simulink model "ANS_GFM_short_term"  (R2021b)
settings: Solver=FixedStepAuto  StartTime=0.0  StopTime=5  FixedStep=Ts  MaxStep=1e-5  RelTol=1e-3
values from neighbouring files (symbols this model uses):
  angle_load = angle(LF.bus(ind_l).Vbus)*180/pi    [init_ANS_GFM_long_term.m]    (also in init_ANS_GFM_short_term.m)
  angleV_LF = Vangle_init/180*pi    [init_ANS_GFM_long_term.m]    (also in init_ANS_GFM_short_term.m)
  awu = 1    [init_ANS_GFM_long_term.m]    (also in init_ANS_GFM_short_term.m)
  C_dc = 1/(Xcdc_pu_or*Zbase_dc_new*100*pi)    [init_ANS_GFM_long_term.m]    (also in init_ANS_GFM_short_term.m)
  C_f = 1/(Xcf_pu_or*Zbase_new*100*pi)    (= 0.013712)    [init_ANS_GFM_long_term.m]    (also in init_ANS_GFM_short_term.m = 0.0141333333333)
  control = 3    [init_ANS_GFM_long_term.m]    (also in init_ANS_GFM_short_term.m = 1)
  D_p = (1/(m_p*w_b))    (= 5209935.26289)    [init_ANS_GFM_long_term.m]    (also in init_ANS_GFM_short_term.m = 5370022.73304)
  Egrid_tmp = 1.054080675694902*400e3    (= 421632.270278)    [init_ANS_GFM_long_term.m]    (also in init_ANS_GFM_short_term.m)
  epsi = 1e-4    (= 0.0001)    [init_ANS_GFM_long_term.m]    (also in init_ANS_GFM_short_term.m)
  eta = m_p*V_m^2    [init_ANS_GFM_long_term.m]    (also in init_ANS_GFM_short_term.m)
  gamma = 2.3    [init_ANS_GFM_long_term.m]    (also in init_ANS_GFM_short_term.m)
  I0_init = [I0_init_a, I0_init_b, I0_init_c]    [init_ANS_GFM_long_term.m]    (also in init_ANS_GFM_short_term.m)
  I_bc = S_bc / (V_bc*sqrt(3))    [init_ANS_GFM_long_term.m]    (also in init_ANS_GFM_short_term.m)
  I_d_int_init = (U_d_int + I_q_int*L_f*w_b - V_d_int - I_d_int*R_f*0)    [init_ANS_GFM_long_term.m]    (also in init_ANS_GFM_short_term.m)
  I_init = [I_init_a, I_init_b, I_init_c]    [init_ANS_GFM_long_term.m]    (also in init_ANS_GFM_short_term.m)
  i_ll = -1.15*(S_bc/Vdc_n)-i_loss_dc    [init_ANS_GFM_long_term.m]    (also in init_ANS_GFM_short_term.m)
  I_max_sat_pu = 1.0 * I_bc *sqrt(2)    [init_ANS_GFM_long_term.m]    (also in init_ANS_GFM_short_term.m)
  I_q_int_init = (U_q_int - I_d_int*L_f*w_b - V_q_int - I_q_int*R_f*0)    [init_ANS_GFM_long_term.m]    (also in init_ANS_GFM_short_term.m)
  i_ul = 1.15*(S_bc/Vdc_n)+i_loss_dc    [init_ANS_GFM_long_term.m]    (also in init_ANS_GFM_short_term.m)
  idppu = 0.95    [init_ANS_GFM_long_term.m]    (also in init_ANS_GFM_short_term.m = 0.92)
  init_dP = -inv(A_pm)*B_pm*dP    [init_ANS_GFM_long_term.m]    (also in init_ANS_GFM_short_term.m)
  init_pm = -inv(A_pm)*B_pm*P_aft    [init_ANS_GFM_long_term.m]    (also in init_ANS_GFM_short_term.m)
  init_tau = -inv(A_tau)*B_tau*idc    [init_ANS_GFM_long_term.m]    (also in init_ANS_GFM_short_term.m)
  J = D_p*tau_f    (= 104198.705258)    [init_ANS_GFM_long_term.m]    (also in init_ANS_GFM_short_term.m = 107400.454661)
  k_dc = eta_1/(Vdc_n*m_p)    [init_ANS_GFM_long_term.m]    (also in init_ANS_GFM_short_term.m)
  K_p = (1/Vdc_n)    [init_ANS_GFM_long_term.m]    (also in init_ANS_GFM_short_term.m)
  K_r = 1/R_dc    [init_ANS_GFM_long_term.m]    (also in init_ANS_GFM_short_term.m)
  Kff_i = 1    [init_ANS_GFM_long_term.m]    (also in init_ANS_GFM_short_term.m)
  Kff_v = 1    [init_ANS_GFM_long_term.m]    (also in init_ANS_GFM_short_term.m)
  Ki_i = (1/n)*1.19    (= 0.0520711785298)    [init_ANS_GFM_long_term.m]    (also in init_ANS_GFM_short_term.m = 0.0505188679245)
  Ki_pll = 4255.3    [init_ANS_GFM_long_term.m]    (also in init_ANS_GFM_short_term.m)
  Ki_v = (n)*1.161022    (= 26.5332227733)    [init_ANS_GFM_long_term.m]    (also in init_ANS_GFM_short_term.m = 27.3485182222)
  ki_v_ac = 2*0.25    (= 0.5)    [init_ANS_GFM_long_term.m]    (also in init_ANS_GFM_short_term.m)
  Kp_i = 0.738891/n    (= 0.032331869895)    [init_ANS_GFM_long_term.m]    (also in init_ANS_GFM_short_term.m = 0.0313680141509)
  Kp_pll = 92    [init_ANS_GFM_long_term.m]    (also in init_ANS_GFM_short_term.m)
  Kp_v = 0.52*n    (= 11.8837333333)    [init_ANS_GFM_long_term.m]    (also in init_ANS_GFM_short_term.m = 12.2488888889)
  kp_v_ac = 0.001    [init_ANS_GFM_long_term.m]    (also in init_ANS_GFM_short_term.m)
  Kpl = 5.0    (= 5)    [init_ANS_GFM_long_term.m]    (also in init_ANS_GFM_short_term.m)
  L1 = cf/sqrt(1+RX^2)*(400e3)^2/Skss/(100*pi)    [init_ANS_GFM_long_term.m]    (also in init_ANS_GFM_short_term.m)
  L_f = Xlf_pu_or*Zbase_new/100/pi    (= 4.37572928821e-06)    [init_ANS_GFM_long_term.m]    (also in init_ANS_GFM_short_term.m = 4.24528301887e-06)
  Lf = 1e6/100/pi    (= 3183.09886184)    [init_ANS_GFM_long_term.m]    (also in init_ANS_GFM_short_term.m = 0.0636619772368)
  m_p = (2*pi*0.5)/(S_bc)    (= 6.10967066042e-10)    [init_ANS_GFM_long_term.m]    (also in init_ANS_GFM_short_term.m = 5.92753330866e-10)
  n = 1/Zb    (= 22.8533333333)    [init_ANS_GFM_long_term.m]    (also in init_ANS_GFM_short_term.m = 23.5555555556)
  P_LF_si = P_LF*S_b    [init_ANS_GFM_long_term.m]    (also in init_ANS_GFM_short_term.m)
  ps = 4440e6/S_bc    (= 0.863477246208)    [init_ANS_GFM_long_term.m]    (also in init_ANS_GFM_short_term.m = 0.837735849057)
  Q_LF_si = Q_LF*S_b    [init_ANS_GFM_long_term.m]    (also in init_ANS_GFM_short_term.m)
  qs = Q_LF*S_b/S_bc    [init_ANS_GFM_long_term.m]    (also in init_ANS_GFM_short_term.m)
  R1 = RX*cf/sqrt(1+RX^2)*(400e3)^2/Skss    [init_ANS_GFM_long_term.m]    (also in init_ANS_GFM_short_term.m)
  R_dc = Rdc_pu_or*Zbase_dc_new    [init_ANS_GFM_long_term.m]    (also in init_ANS_GFM_short_term.m)
  R_f = Rf_pu_or*Zbase_new    (= 2.18786464411e-05)    [init_ANS_GFM_long_term.m]    (also in init_ANS_GFM_short_term.m = 2.12264150943e-05)
  Rf = 1e6    (= 1000000)    [init_ANS_GFM_long_term.m]    (also in init_ANS_GFM_short_term.m = 20)
  S_bc = 5142e6    (= 5142000000)    [init_ANS_GFM_long_term.m]    (also in init_ANS_GFM_short_term.m = 5300000000)
  sat_select = 3    [init_ANS_GFM_long_term.m]    (also in init_ANS_GFM_short_term.m)
  SECM = 3    [init_ANS_GFM_long_term.m]    (also in init_ANS_GFM_short_term.m = 1)
  share_i_load = 1.0    (= 1)    [init_ANS_GFM_long_term.m]    (also in init_ANS_GFM_short_term.m)
  T_en = -0.5    [init_ANS_GFM_long_term.m]    (also in init_ANS_GFM_short_term.m)
  T_off = T_on + 0.1    (= 0.2)    [init_ANS_GFM_long_term.m]    (also in init_ANS_GFM_short_term.m)
  T_on = 0.1    [init_ANS_GFM_long_term.m]    (also in init_ANS_GFM_short_term.m)
  Ts = 2e-6    (= 2e-06)    [init_ANS_GFM_long_term.m]    (also in init_ANS_GFM_short_term.m = 1e-06)
  U_init = [Umag_init_a, Umag_init_b, Umag_init_c]    [init_ANS_GFM_long_term.m]    (also in init_ANS_GFM_short_term.m)
  Uangle_init = angle(V_LF_VSC)*180/pi    [init_ANS_GFM_long_term.m]    (also in init_ANS_GFM_short_term.m)
  Umag_init = abs(V_LF_VSC)*V_bc*sqrt(2/3)    [init_ANS_GFM_long_term.m]    (also in init_ANS_GFM_short_term.m)
  V1_rms = 15e3    (= 15000)    [init_ANS_GFM_long_term.m]    (also in init_ANS_GFM_short_term.m)
  V_d_int = abs(V_LF)*V_bc*sqrt(2/3)    [init_ANS_GFM_long_term.m]    (also in init_ANS_GFM_short_term.m)
  V_d_int_init = (I_d_int + V_q_int*C_f*w_b - I0_d_int)    [init_ANS_GFM_long_term.m]    (also in init_ANS_GFM_short_term.m)
  V_init = [V_init_a, V_init_b, V_init_c]    [init_ANS_GFM_long_term.m]    (also in init_ANS_GFM_short_term.m)
  V_m = sqrt(2/3)*V_bc    [init_ANS_GFM_long_term.m]    (also in init_ANS_GFM_short_term.m)
  V_q_int_init = (I_q_int - V_d_int*C_f*w_b - I0_q_int)    [init_ANS_GFM_long_term.m]    (also in init_ANS_GFM_short_term.m)
  Vdc_n = 3*V_m    [init_ANS_GFM_long_term.m]    (also in init_ANS_GFM_short_term.m)
  Vref = V_LF_mag*V_m    [init_ANS_GFM_long_term.m]    (also in init_ANS_GFM_short_term.m)
  w_b = 2*pi*f_b    (= 314.159265359)    [init_ANS_GFM_long_term.m]    (also in init_ANS_GFM_short_term.m)
  w_f = 2*pi*5    (= 31.4159265359)    [init_ANS_GFM_long_term.m]    (also in init_ANS_GFM_short_term.m)
  Zbase_new = V1_rms^2/S_bc    (= 0.0437572928821)    [init_ANS_GFM_long_term.m]    (also in init_ANS_GFM_short_term.m = 0.0424528301887)
undefined symbols (not defined in the file or in its folder): A_pm, A_tau, B_pm, B_tau, C_pm, C_tau, D_pm, D_tau, find_system, idq0_init, Pm, sm_init, v_d, v_q, Ve
libraries: spsBreakerLib x270, spsGroundLib x21, spsThreePhaseSeriesRLCBranchLib x12, spsabctodq0Lib x11, simulink x9, spsEdgeDetectorLib x8, spsThreePhaseVIMeasurementLib x7, spsLoadFlowBusLib x7, spsSeriesRLCBranchLib x6, spsControlledVoltageSourceLib x6, spsCurrentMeasurementLib x6, spsVoltageMeasurementLib x6
(part 4 of 7)

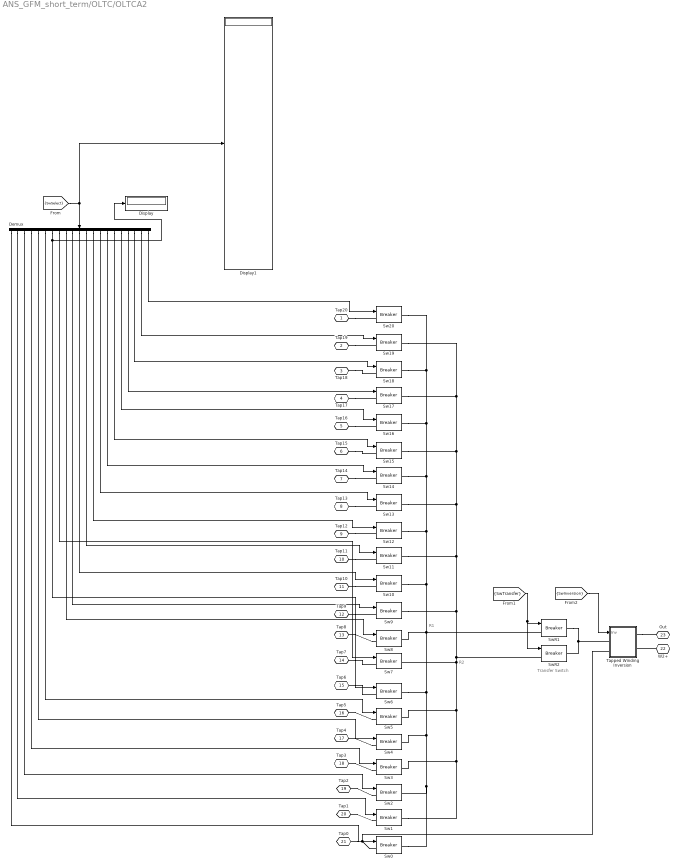
== system ANS_GFM_short_term/OLTC/OLTCA2 ==
  note: R2
  note: R1
  note: Transfer Switch
  Demux : Demux  Outputs=21
      settings: DisplayOption=none
  Display : Display
  Display1 : Display
  "Sw0 " : spsBreakerLib/Breaker  InitialState=InitialStates(1)  SwitchingTimes="[ 1/60  5/60 ]"  External=on  BreakerResistance=Rswitch  SnubberResistance=1e8  SnubberCapacitance=inf  Measurements=None  MoreParameters=off  NoBreakLoop=off
      settings: SourceProductBaseCode=PS
  "Sw1 " : spsBreakerLib/Breaker  InitialState=InitialStates(2)  SwitchingTimes="[ 1/60  5/60 ]"  External=on  BreakerResistance=Rswitch  SnubberResistance=1e8  SnubberCapacitance=inf  Measurements=None  MoreParameters=off  NoBreakLoop=off
      settings: SourceProductBaseCode=PS
  Sw10 : spsBreakerLib/Breaker  InitialState=InitialStates(11)  SwitchingTimes="[ 1/60  5/60 ]"  External=on  BreakerResistance=Rswitch  SnubberResistance=1e8  SnubberCapacitance=inf  Measurements=None  MoreParameters=off  NoBreakLoop=off
      settings: SourceProductBaseCode=PS
  Sw11 : spsBreakerLib/Breaker  InitialState=InitialStates(12)  SwitchingTimes="[ 1/60  5/60 ]"  External=on  BreakerResistance=Rswitch  SnubberResistance=1e8  SnubberCapacitance=inf  Measurements=None  MoreParameters=off  NoBreakLoop=off
      settings: SourceProductBaseCode=PS
  Sw12 : spsBreakerLib/Breaker  InitialState=InitialStates(13)  SwitchingTimes="[ 1/60  5/60 ]"  External=on  BreakerResistance=Rswitch  SnubberResistance=1e8  SnubberCapacitance=inf  Measurements=None  MoreParameters=off  NoBreakLoop=off
      settings: SourceProductBaseCode=PS
  Sw13 : spsBreakerLib/Breaker  InitialState=InitialStates(14)  SwitchingTimes="[ 1/60  5/60 ]"  External=on  BreakerResistance=Rswitch  SnubberResistance=1e8  SnubberCapacitance=inf  Measurements=None  MoreParameters=off  NoBreakLoop=off
      settings: SourceProductBaseCode=PS
  Sw14 : spsBreakerLib/Breaker  InitialState=InitialStates(15)  SwitchingTimes="[ 1/60  5/60 ]"  External=on  BreakerResistance=Rswitch  SnubberResistance=1e8  SnubberCapacitance=inf  Measurements=None  MoreParameters=off  NoBreakLoop=off
      settings: SourceProductBaseCode=PS
  Sw15 : spsBreakerLib/Breaker  InitialState=InitialStates(16)  SwitchingTimes="[ 1/60  5/60 ]"  External=on  BreakerResistance=Rswitch  SnubberResistance=1e8  SnubberCapacitance=inf  Measurements=None  MoreParameters=off  NoBreakLoop=off
      settings: SourceProductBaseCode=PS
  Sw16 : spsBreakerLib/Breaker  InitialState=InitialStates(17)  SwitchingTimes="[ 1/60  5/60 ]"  External=on  BreakerResistance=Rswitch  SnubberResistance=1e8  SnubberCapacitance=inf  Measurements=None  MoreParameters=off  NoBreakLoop=off
      settings: SourceProductBaseCode=PS
  Sw17 : spsBreakerLib/Breaker  InitialState=InitialStates(18)  SwitchingTimes="[ 1/60  5/60 ]"  External=on  BreakerResistance=Rswitch  SnubberResistance=1e8  SnubberCapacitance=inf  Measurements=None  MoreParameters=off  NoBreakLoop=off
      settings: SourceProductBaseCode=PS
  Sw18 : spsBreakerLib/Breaker  InitialState=InitialStates(19)  SwitchingTimes="[ 1/60  5/60 ]"  External=on  BreakerResistance=Rswitch  SnubberResistance=1e8  SnubberCapacitance=inf  Measurements=None  MoreParameters=off  NoBreakLoop=off
      settings: SourceProductBaseCode=PS
  Sw19 : spsBreakerLib/Breaker  InitialState=InitialStates(20)  SwitchingTimes="[ 1/60  5/60 ]"  External=on  BreakerResistance=Rswitch  SnubberResistance=1e8  SnubberCapacitance=inf  Measurements=None  MoreParameters=off  NoBreakLoop=off
      settings: SourceProductBaseCode=PS
  "Sw2 " : spsBreakerLib/Breaker  InitialState=InitialStates(3)  SwitchingTimes="[ 1/60  5/60 ]"  External=on  BreakerResistance=Rswitch  SnubberResistance=1e8  SnubberCapacitance=inf  Measurements=None  MoreParameters=off  NoBreakLoop=off
      settings: SourceProductBaseCode=PS
  Sw20 : spsBreakerLib/Breaker  InitialState=InitialStates(21)  SwitchingTimes="[ 1/60  5/60 ]"  External=on  BreakerResistance=Rswitch  SnubberResistance=Rsnubber  SnubberCapacitance=inf  Measurements=None  MoreParameters=off  NoBreakLoop=off
      settings: SourceProductBaseCode=PS
  "Sw3 " : spsBreakerLib/Breaker  InitialState=InitialStates(4)  SwitchingTimes="[ 1/60  5/60 ]"  External=on  BreakerResistance=Rswitch  SnubberResistance=1e8  SnubberCapacitance=inf  Measurements=None  MoreParameters=off  NoBreakLoop=off
      settings: SourceProductBaseCode=PS
  "Sw4 " : spsBreakerLib/Breaker  InitialState=InitialStates(5)  SwitchingTimes="[ 1/60  5/60 ]"  External=on  BreakerResistance=Rswitch  SnubberResistance=1e8  SnubberCapacitance=inf  Measurements=None  MoreParameters=off  NoBreakLoop=off
      settings: SourceProductBaseCode=PS
  "Sw5 " : spsBreakerLib/Breaker  InitialState=InitialStates(6)  SwitchingTimes="[ 1/60  5/60 ]"  External=on  BreakerResistance=Rswitch  SnubberResistance=1e8  SnubberCapacitance=inf  Measurements=None  MoreParameters=off  NoBreakLoop=off
      settings: SourceProductBaseCode=PS
  "Sw6 " : spsBreakerLib/Breaker  InitialState=InitialStates(7)  SwitchingTimes="[ 1/60  5/60 ]"  External=on  BreakerResistance=Rswitch  SnubberResistance=1e8  SnubberCapacitance=inf  Measurements=None  MoreParameters=off  NoBreakLoop=off
      settings: SourceProductBaseCode=PS
  "Sw7 " : spsBreakerLib/Breaker  InitialState=InitialStates(8)  SwitchingTimes="[ 1/60  5/60 ]"  External=on  BreakerResistance=Rswitch  SnubberResistance=1e8  SnubberCapacitance=inf  Measurements=None  MoreParameters=off  NoBreakLoop=off
      settings: SourceProductBaseCode=PS
  "Sw8 " : spsBreakerLib/Breaker  InitialState=InitialStates(9)  SwitchingTimes="[ 1/60  5/60 ]"  External=on  BreakerResistance=Rswitch  SnubberResistance=1e8  SnubberCapacitance=inf  Measurements=None  MoreParameters=off  NoBreakLoop=off
      settings: SourceProductBaseCode=PS
  Sw9 : spsBreakerLib/Breaker  InitialState=InitialStates(10)  SwitchingTimes="[ 1/60  5/60 ]"  External=on  BreakerResistance=Rswitch  SnubberResistance=1e8  SnubberCapacitance=inf  Measurements=None  MoreParameters=off  NoBreakLoop=off
      settings: SourceProductBaseCode=PS
  SwR1 : spsBreakerLib/Breaker  InitialState=1  SwitchingTimes="[ 1/60  5/60 ]"  External=on  BreakerResistance=Rswitch  SnubberResistance=Rtransfer  SnubberCapacitance=inf  Measurements=None  MoreParameters=off  NoBreakLoop=off
      settings: SourceProductBaseCode=PS
  SwR2 : spsBreakerLib/Breaker  InitialState=1  SwitchingTimes="[ 1/60  5/60 ]"  External=on  BreakerResistance=Rswitch  SnubberResistance=Rtransfer  SnubberCapacitance=inf  Measurements=None  MoreParameters=off  NoBreakLoop=off
      settings: SourceProductBaseCode=PS
  Tapped Winding Inversion : Subsystem
  Tap20 : PMIOPort  Side=Right
  Tap19 : PMIOPort  Port=2  Side=Right
  Tap18 : PMIOPort  Port=3  Side=Right
  Tap17 : PMIOPort  Port=4  Side=Right
  Tap16 : PMIOPort  Port=5  Side=Right
  Tap15 : PMIOPort  Port=6  Side=Right
  Tap14 : PMIOPort  Port=7  Side=Right
  Tap13 : PMIOPort  Port=8  Side=Right
  Tap12 : PMIOPort  Port=9  Side=Right
  Tap11 : PMIOPort  Port=10  Side=Right
  Tap10 : PMIOPort  Port=11  Side=Right
  Tap9 : PMIOPort  Port=12  Side=Right
  Tap8 : PMIOPort  Port=13  Side=Right
  Tap7 : PMIOPort  Port=14  Side=Right
  Tap6 : PMIOPort  Port=15  Side=Right
  Tap5 : PMIOPort  Port=16  Side=Right
  Tap4 : PMIOPort  Port=17  Side=Right
  Tap3 : PMIOPort  Port=18  Side=Right
  Tap2 : PMIOPort  Port=19  Side=Right
  Tap1 : PMIOPort  Port=20  Side=Right
  Tap0 : PMIOPort  Port=21  Side=Right
  W2+ : PMIOPort  Port=22  Side=Right
  Out : PMIOPort  Port=23  Side=Left
  wires:
  Demux/9 -> "Sw8 "/1
  Demux/8 -> "Sw7 "/1
  Demux/7 -> Display/1, "Sw6 "/1
  Demux/6 -> "Sw5 "/1
  Demux/5 -> "Sw4 "/1
  Demux/4 -> "Sw3 "/1
  Demux/3 -> "Sw2 "/1
  Demux/2 -> "Sw1 "/1
  Demux/1 -> "Sw0 "/1
  [SwInversion] -> Tapped Winding Inversion/1(Inv)
  [SwTransfer] -> SwR2/1, SwR1/1
  [SwSelect] -> Demux/1, Display1/1
  Demux/10 -> Sw9/1
  Demux/11 -> Sw10/1
  Demux/12 -> Sw11/1
  Demux/13 -> Sw12/1
  Demux/14 -> Sw13/1
  Demux/15 -> Sw14/1
  Demux/16 -> Sw15/1
  Demux/17 -> Sw16/1
  Demux/18 -> Sw17/1
  Demux/19 -> Sw18/1
  Demux/20 -> Sw19/1
  Demux/21 -> Sw20/1
  connections:
  "Sw0 "/LConn1 -- Tap0/RConn1 -- Tapped Winding Inversion/LConn2
  Tap1/RConn1 -- "Sw1 "/LConn1
  Tap2/RConn1 -- "Sw2 "/LConn1
  Tap6/RConn1 -- "Sw6 "/LConn1
  Tap4/RConn1 -- "Sw4 "/LConn1
  Tap5/RConn1 -- "Sw5 "/LConn1
  SwR1/RConn1 -- Tapped Winding Inversion/LConn1 -- SwR2/RConn1
  Sw19/RConn1 -- Sw17/RConn1 -- Sw15/RConn1 -- Sw13/RConn1 -- Sw11/RConn1 -- Sw9/RConn1 -- SwR2/LConn1 -- "Sw5 "/RConn1 -- "Sw3 "/RConn1 -- "Sw1 "/RConn1 -- "Sw7 "/RConn1
  Tapped Winding Inversion/RConn1 -- Out/RConn1
  W2+/RConn1 -- Tapped Winding Inversion/RConn2
  "Sw6 "/RConn1 -- "Sw4 "/RConn1 -- "Sw2 "/RConn1 -- "Sw0 "/RConn1 -- Sw20/RConn1 -- Sw18/RConn1 -- Sw16/RConn1 -- Sw14/RConn1 -- Sw12/RConn1 -- Sw10/RConn1 -- "Sw8 "/RConn1 -- SwR1/LConn1
  Tap3/RConn1 -- "Sw3 "/LConn1
  Tap8/RConn1 -- "Sw8 "/LConn1
  Tap7/RConn1 -- "Sw7 "/LConn1
  Tap9/RConn1 -- Sw9/LConn1
  Tap10/RConn1 -- Sw10/LConn1
  Tap11/RConn1 -- Sw11/LConn1
  Tap13/RConn1 -- Sw13/LConn1
  Tap12/RConn1 -- Sw12/LConn1
  Tap14/RConn1 -- Sw14/LConn1
  Tap15/RConn1 -- Sw15/LConn1
  Tap16/RConn1 -- Sw16/LConn1
  Tap17/RConn1 -- Sw17/LConn1
  Tap18/RConn1 -- Sw18/LConn1
  Tap19/RConn1 -- Sw19/LConn1
  Tap20/RConn1 -- Sw20/LConn1

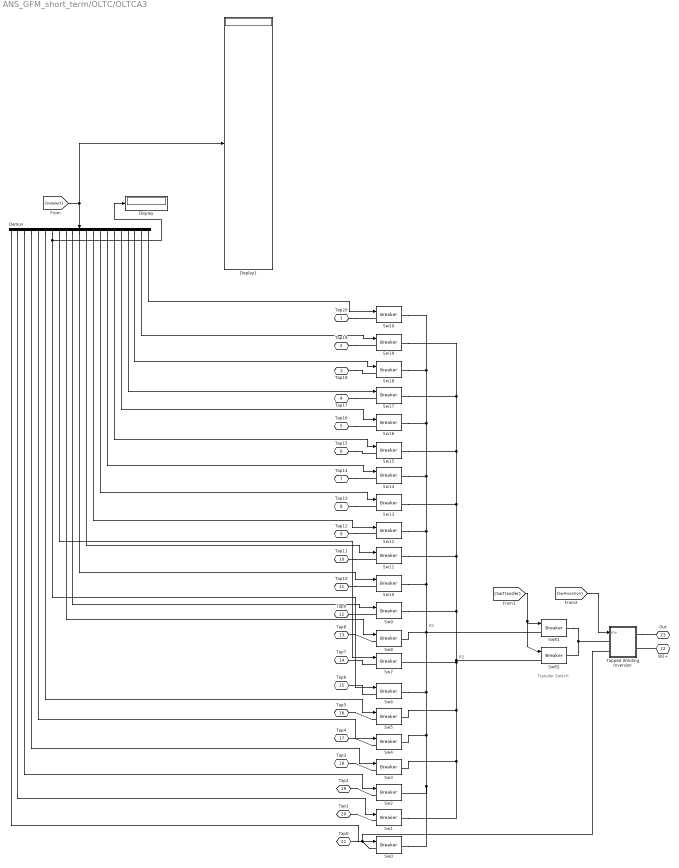
== system ANS_GFM_short_term/OLTC/OLTCA3 ==
  note: R2
  note: R1
  note: Transfer Switch
  Demux : Demux  Outputs=21
      settings: DisplayOption=none
  Display : Display
  Display1 : Display
  "Sw0 " : spsBreakerLib/Breaker  InitialState=InitialStates(1)  SwitchingTimes="[ 1/60  5/60 ]"  External=on  BreakerResistance=1e-8  SnubberResistance=1e8  SnubberCapacitance=inf  Measurements=None  MoreParameters=off  NoBreakLoop=off
      settings: SourceProductBaseCode=PS
  "Sw1 " : spsBreakerLib/Breaker  InitialState=InitialStates(2)  SwitchingTimes="[ 1/60  5/60 ]"  External=on  BreakerResistance=1e-8  SnubberResistance=1e8  SnubberCapacitance=inf  Measurements=None  MoreParameters=off  NoBreakLoop=off
      settings: SourceProductBaseCode=PS
  Sw10 : spsBreakerLib/Breaker  InitialState=InitialStates(11)  SwitchingTimes="[ 1/60  5/60 ]"  External=on  BreakerResistance=1e-8  SnubberResistance=1e8  SnubberCapacitance=inf  Measurements=None  MoreParameters=off  NoBreakLoop=off
      settings: SourceProductBaseCode=PS
  Sw11 : spsBreakerLib/Breaker  InitialState=InitialStates(12)  SwitchingTimes="[ 1/60  5/60 ]"  External=on  BreakerResistance=1e-8  SnubberResistance=1e8  SnubberCapacitance=inf  Measurements=None  MoreParameters=off  NoBreakLoop=off
      settings: SourceProductBaseCode=PS
  Sw12 : spsBreakerLib/Breaker  InitialState=InitialStates(13)  SwitchingTimes="[ 1/60  5/60 ]"  External=on  BreakerResistance=1e-8  SnubberResistance=1e8  SnubberCapacitance=inf  Measurements=None  MoreParameters=off  NoBreakLoop=off
      settings: SourceProductBaseCode=PS
  Sw13 : spsBreakerLib/Breaker  InitialState=InitialStates(14)  SwitchingTimes="[ 1/60  5/60 ]"  External=on  BreakerResistance=1e-8  SnubberResistance=1e8  SnubberCapacitance=inf  Measurements=None  MoreParameters=off  NoBreakLoop=off
      settings: SourceProductBaseCode=PS
  Sw14 : spsBreakerLib/Breaker  InitialState=InitialStates(15)  SwitchingTimes="[ 1/60  5/60 ]"  External=on  BreakerResistance=1e-8  SnubberResistance=1e8  SnubberCapacitance=inf  Measurements=None  MoreParameters=off  NoBreakLoop=off
      settings: SourceProductBaseCode=PS
  Sw15 : spsBreakerLib/Breaker  InitialState=InitialStates(16)  SwitchingTimes="[ 1/60  5/60 ]"  External=on  BreakerResistance=1e-8  SnubberResistance=1e8  SnubberCapacitance=inf  Measurements=None  MoreParameters=off  NoBreakLoop=off
      settings: SourceProductBaseCode=PS
  Sw16 : spsBreakerLib/Breaker  InitialState=InitialStates(17)  SwitchingTimes="[ 1/60  5/60 ]"  External=on  BreakerResistance=1e-8  SnubberResistance=1e8  SnubberCapacitance=inf  Measurements=None  MoreParameters=off  NoBreakLoop=off
      settings: SourceProductBaseCode=PS
  Sw17 : spsBreakerLib/Breaker  InitialState=InitialStates(18)  SwitchingTimes="[ 1/60  5/60 ]"  External=on  BreakerResistance=1e-8  SnubberResistance=1e8  SnubberCapacitance=inf  Measurements=None  MoreParameters=off  NoBreakLoop=off
      settings: SourceProductBaseCode=PS
  Sw18 : spsBreakerLib/Breaker  InitialState=InitialStates(19)  SwitchingTimes="[ 1/60  5/60 ]"  External=on  BreakerResistance=1e-8  SnubberResistance=1e8  SnubberCapacitance=inf  Measurements=None  MoreParameters=off  NoBreakLoop=off
      settings: SourceProductBaseCode=PS
  Sw19 : spsBreakerLib/Breaker  InitialState=InitialStates(20)  SwitchingTimes="[ 1/60  5/60 ]"  External=on  BreakerResistance=1e-8  SnubberResistance=1e8  SnubberCapacitance=inf  Measurements=None  MoreParameters=off  NoBreakLoop=off
      settings: SourceProductBaseCode=PS
  "Sw2 " : spsBreakerLib/Breaker  InitialState=InitialStates(3)  SwitchingTimes="[ 1/60  5/60 ]"  External=on  BreakerResistance=1e-8  SnubberResistance=1e8  SnubberCapacitance=inf  Measurements=None  MoreParameters=off  NoBreakLoop=off
      settings: SourceProductBaseCode=PS
  Sw20 : spsBreakerLib/Breaker  InitialState=InitialStates(21)  SwitchingTimes="[ 1/60  5/60 ]"  External=on  BreakerResistance=1e-8  SnubberResistance=1e8  SnubberCapacitance=inf  Measurements=None  MoreParameters=off  NoBreakLoop=off
      settings: SourceProductBaseCode=PS
  "Sw3 " : spsBreakerLib/Breaker  InitialState=InitialStates(4)  SwitchingTimes="[ 1/60  5/60 ]"  External=on  BreakerResistance=1e-8  SnubberResistance=1e8  SnubberCapacitance=inf  Measurements=None  MoreParameters=off  NoBreakLoop=off
      settings: SourceProductBaseCode=PS
  "Sw4 " : spsBreakerLib/Breaker  InitialState=InitialStates(5)  SwitchingTimes="[ 1/60  5/60 ]"  External=on  BreakerResistance=1e-8  SnubberResistance=1e8  SnubberCapacitance=inf  Measurements=None  MoreParameters=off  NoBreakLoop=off
      settings: SourceProductBaseCode=PS
  "Sw5 " : spsBreakerLib/Breaker  InitialState=InitialStates(6)  SwitchingTimes="[ 1/60  5/60 ]"  External=on  BreakerResistance=1e-8  SnubberResistance=1e8  SnubberCapacitance=inf  Measurements=None  MoreParameters=off  NoBreakLoop=off
      settings: SourceProductBaseCode=PS
  "Sw6 " : spsBreakerLib/Breaker  InitialState=InitialStates(7)  SwitchingTimes="[ 1/60  5/60 ]"  External=on  BreakerResistance=1e-8  SnubberResistance=1e8  SnubberCapacitance=inf  Measurements=None  MoreParameters=off  NoBreakLoop=off
      settings: SourceProductBaseCode=PS
  "Sw7 " : spsBreakerLib/Breaker  InitialState=InitialStates(8)  SwitchingTimes="[ 1/60  5/60 ]"  External=on  BreakerResistance=1e-8  SnubberResistance=1e8  SnubberCapacitance=inf  Measurements=None  MoreParameters=off  NoBreakLoop=off
      settings: SourceProductBaseCode=PS
  "Sw8 " : spsBreakerLib/Breaker  InitialState=InitialStates(9)  SwitchingTimes="[ 1/60  5/60 ]"  External=on  BreakerResistance=1e-8  SnubberResistance=1e8  SnubberCapacitance=inf  Measurements=None  MoreParameters=off  NoBreakLoop=off
      settings: SourceProductBaseCode=PS
  Sw9 : spsBreakerLib/Breaker  InitialState=InitialStates(10)  SwitchingTimes="[ 1/60  5/60 ]"  External=on  BreakerResistance=1e-8  SnubberResistance=1e8  SnubberCapacitance=inf  Measurements=None  MoreParameters=off  NoBreakLoop=off
      settings: SourceProductBaseCode=PS
  SwR1 : spsBreakerLib/Breaker  InitialState=1  SwitchingTimes="[ 1/60  5/60 ]"  External=on  BreakerResistance=1e-8  SnubberResistance=Rtransfer  SnubberCapacitance=inf  Measurements=None  MoreParameters=off  NoBreakLoop=off
      settings: SourceProductBaseCode=PS
  SwR2 : spsBreakerLib/Breaker  InitialState=1  SwitchingTimes="[ 1/60  5/60 ]"  External=on  BreakerResistance=1e-8  SnubberResistance=Rtransfer  SnubberCapacitance=inf  Measurements=None  MoreParameters=off  NoBreakLoop=off
      settings: SourceProductBaseCode=PS
  Tapped Winding Inversion : Subsystem
  Tap20 : PMIOPort  Side=Right
  Tap19 : PMIOPort  Port=2  Side=Right
  Tap18 : PMIOPort  Port=3  Side=Right
  Tap17 : PMIOPort  Port=4  Side=Right
  Tap16 : PMIOPort  Port=5  Side=Right
  Tap15 : PMIOPort  Port=6  Side=Right
  Tap14 : PMIOPort  Port=7  Side=Right
  Tap13 : PMIOPort  Port=8  Side=Right
  Tap12 : PMIOPort  Port=9  Side=Right
  Tap11 : PMIOPort  Port=10  Side=Right
  Tap10 : PMIOPort  Port=11  Side=Right
  Tap9 : PMIOPort  Port=12  Side=Right
  Tap8 : PMIOPort  Port=13  Side=Right
  Tap7 : PMIOPort  Port=14  Side=Right
  Tap6 : PMIOPort  Port=15  Side=Right
  Tap5 : PMIOPort  Port=16  Side=Right
  Tap4 : PMIOPort  Port=17  Side=Right
  Tap3 : PMIOPort  Port=18  Side=Right
  Tap2 : PMIOPort  Port=19  Side=Right
  Tap1 : PMIOPort  Port=20  Side=Right
  Tap0 : PMIOPort  Port=21  Side=Right
  W2+ : PMIOPort  Port=22  Side=Right
  Out : PMIOPort  Port=23  Side=Left
  wires:
  Demux/9 -> "Sw8 "/1
  Demux/8 -> "Sw7 "/1
  Demux/7 -> Display/1, "Sw6 "/1
  Demux/6 -> "Sw5 "/1
  Demux/5 -> "Sw4 "/1
  Demux/4 -> "Sw3 "/1
  Demux/3 -> "Sw2 "/1
  Demux/2 -> "Sw1 "/1
  Demux/1 -> "Sw0 "/1
  [SwInversion] -> Tapped Winding Inversion/1(Inv)
  [SwTransfer] -> SwR2/1, SwR1/1
  [SwSelect] -> Demux/1, Display1/1
  Demux/10 -> Sw9/1
  Demux/11 -> Sw10/1
  Demux/12 -> Sw11/1
  Demux/13 -> Sw12/1
  Demux/14 -> Sw13/1
  Demux/15 -> Sw14/1
  Demux/16 -> Sw15/1
  Demux/17 -> Sw16/1
  Demux/18 -> Sw17/1
  Demux/19 -> Sw18/1
  Demux/20 -> Sw19/1
  Demux/21 -> Sw20/1
  connections:
  "Sw0 "/LConn1 -- Tap0/RConn1 -- Tapped Winding Inversion/LConn2
  Tap1/RConn1 -- "Sw1 "/LConn1
  Tap2/RConn1 -- "Sw2 "/LConn1
  Tap6/RConn1 -- "Sw6 "/LConn1
  Tap4/RConn1 -- "Sw4 "/LConn1
  Tap5/RConn1 -- "Sw5 "/LConn1
  SwR1/RConn1 -- Tapped Winding Inversion/LConn1 -- SwR2/RConn1
  Sw19/RConn1 -- Sw17/RConn1 -- Sw15/RConn1 -- Sw13/RConn1 -- Sw11/RConn1 -- Sw9/RConn1 -- SwR2/LConn1 -- "Sw5 "/RConn1 -- "Sw3 "/RConn1 -- "Sw1 "/RConn1 -- "Sw7 "/RConn1
  Tapped Winding Inversion/RConn1 -- Out/RConn1
  W2+/RConn1 -- Tapped Winding Inversion/RConn2
  "Sw6 "/RConn1 -- "Sw4 "/RConn1 -- "Sw2 "/RConn1 -- "Sw0 "/RConn1 -- Sw20/RConn1 -- Sw18/RConn1 -- Sw16/RConn1 -- Sw14/RConn1 -- Sw12/RConn1 -- Sw10/RConn1 -- "Sw8 "/RConn1 -- SwR1/LConn1
  Tap3/RConn1 -- "Sw3 "/LConn1
  Tap8/RConn1 -- "Sw8 "/LConn1
  Tap7/RConn1 -- "Sw7 "/LConn1
  Tap9/RConn1 -- Sw9/LConn1
  Tap10/RConn1 -- Sw10/LConn1
  Tap11/RConn1 -- Sw11/LConn1
  Tap13/RConn1 -- Sw13/LConn1
  Tap12/RConn1 -- Sw12/LConn1
  Tap14/RConn1 -- Sw14/LConn1
  Tap15/RConn1 -- Sw15/LConn1
  Tap16/RConn1 -- Sw16/LConn1
  Tap17/RConn1 -- Sw17/LConn1
  Tap18/RConn1 -- Sw18/LConn1
  Tap19/RConn1 -- Sw19/LConn1
  Tap20/RConn1 -- Sw20/LConn1

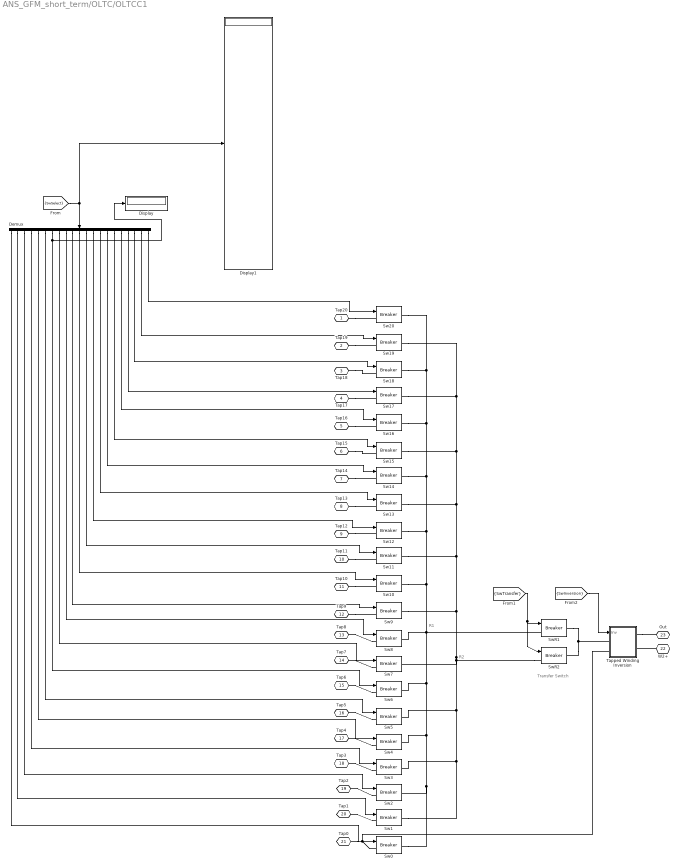
== system ANS_GFM_short_term/OLTC/OLTCC1 ==
  note: R2
  note: R1
  note: Transfer Switch
  Demux : Demux  Outputs=21
      settings: DisplayOption=none
  Display : Display
  Display1 : Display
  "Sw0 " : spsBreakerLib/Breaker  InitialState=InitialStates(1)  SwitchingTimes="[ 1/60  5/60 ]"  External=on  BreakerResistance=1e-6  SnubberResistance=1e8  SnubberCapacitance=inf  Measurements=None  MoreParameters=off  NoBreakLoop=off
      settings: SourceProductBaseCode=PS
  "Sw1 " : spsBreakerLib/Breaker  InitialState=InitialStates(2)  SwitchingTimes="[ 1/60  5/60 ]"  External=on  BreakerResistance=1e-4  SnubberResistance=1e6  SnubberCapacitance=inf  Measurements=None  MoreParameters=off  NoBreakLoop=off
      settings: SourceProductBaseCode=PS
  Sw10 : spsBreakerLib/Breaker  InitialState=InitialStates(11)  SwitchingTimes="[ 1/60  5/60 ]"  External=on  BreakerResistance=1e-6  SnubberResistance=1e8  SnubberCapacitance=inf  Measurements=None  MoreParameters=off  NoBreakLoop=off
      settings: SourceProductBaseCode=PS
  Sw11 : spsBreakerLib/Breaker  InitialState=InitialStates(12)  SwitchingTimes="[ 1/60  5/60 ]"  External=on  BreakerResistance=1e-6  SnubberResistance=1e8  SnubberCapacitance=inf  Measurements=None  MoreParameters=off  NoBreakLoop=off
      settings: SourceProductBaseCode=PS
  Sw12 : spsBreakerLib/Breaker  InitialState=InitialStates(13)  SwitchingTimes="[ 1/60  5/60 ]"  External=on  BreakerResistance=1e-6  SnubberResistance=1e8  SnubberCapacitance=inf  Measurements=None  MoreParameters=off  NoBreakLoop=off
      settings: SourceProductBaseCode=PS
  Sw13 : spsBreakerLib/Breaker  InitialState=InitialStates(14)  SwitchingTimes="[ 1/60  5/60 ]"  External=on  BreakerResistance=1e-4  SnubberResistance=1e6  SnubberCapacitance=inf  Measurements=None  MoreParameters=off  NoBreakLoop=off
      settings: SourceProductBaseCode=PS
  Sw14 : spsBreakerLib/Breaker  InitialState=InitialStates(15)  SwitchingTimes="[ 1/60  5/60 ]"  External=on  BreakerResistance=1e-4  SnubberResistance=1e6  SnubberCapacitance=inf  Measurements=None  MoreParameters=off  NoBreakLoop=off
      settings: SourceProductBaseCode=PS
  Sw15 : spsBreakerLib/Breaker  InitialState=InitialStates(16)  SwitchingTimes="[ 1/60  5/60 ]"  External=on  BreakerResistance=1e-4  SnubberResistance=1e6  SnubberCapacitance=inf  Measurements=None  MoreParameters=off  NoBreakLoop=off
      settings: SourceProductBaseCode=PS
  Sw16 : spsBreakerLib/Breaker  InitialState=InitialStates(17)  SwitchingTimes="[ 1/60  5/60 ]"  External=on  BreakerResistance=1e-4  SnubberResistance=1e6  SnubberCapacitance=inf  Measurements=None  MoreParameters=off  NoBreakLoop=off
      settings: SourceProductBaseCode=PS
  Sw17 : spsBreakerLib/Breaker  InitialState=InitialStates(18)  SwitchingTimes="[ 1/60  5/60 ]"  External=on  BreakerResistance=1e-4  SnubberResistance=1e6  SnubberCapacitance=inf  Measurements=None  MoreParameters=off  NoBreakLoop=off
      settings: SourceProductBaseCode=PS
  Sw18 : spsBreakerLib/Breaker  InitialState=InitialStates(19)  SwitchingTimes="[ 1/60  5/60 ]"  External=on  BreakerResistance=1e-4  SnubberResistance=1e6  SnubberCapacitance=inf  Measurements=None  MoreParameters=off  NoBreakLoop=off
      settings: SourceProductBaseCode=PS
  Sw19 : spsBreakerLib/Breaker  InitialState=InitialStates(20)  SwitchingTimes="[ 1/60  5/60 ]"  External=on  BreakerResistance=1e-4  SnubberResistance=1e6  SnubberCapacitance=inf  Measurements=None  MoreParameters=off  NoBreakLoop=off
      settings: SourceProductBaseCode=PS
  "Sw2 " : spsBreakerLib/Breaker  InitialState=InitialStates(3)  SwitchingTimes="[ 1/60  5/60 ]"  External=on  BreakerResistance=1e-4  SnubberResistance=1e6  SnubberCapacitance=inf  Measurements=None  MoreParameters=off  NoBreakLoop=off
      settings: SourceProductBaseCode=PS
  Sw20 : spsBreakerLib/Breaker  InitialState=InitialStates(21)  SwitchingTimes="[ 1/60  5/60 ]"  External=on  BreakerResistance=1e-4  SnubberResistance=1e6  SnubberCapacitance=inf  Measurements=None  MoreParameters=off  NoBreakLoop=off
      settings: SourceProductBaseCode=PS
  "Sw3 " : spsBreakerLib/Breaker  InitialState=InitialStates(4)  SwitchingTimes="[ 1/60  5/60 ]"  External=on  BreakerResistance=1e-4  SnubberResistance=1e6  SnubberCapacitance=inf  Measurements=None  MoreParameters=off  NoBreakLoop=off
      settings: SourceProductBaseCode=PS
  "Sw4 " : spsBreakerLib/Breaker  InitialState=InitialStates(5)  SwitchingTimes="[ 1/60  5/60 ]"  External=on  BreakerResistance=1e-4  SnubberResistance=1e6  SnubberCapacitance=inf  Measurements=None  MoreParameters=off  NoBreakLoop=off
      settings: SourceProductBaseCode=PS
  "Sw5 " : spsBreakerLib/Breaker  InitialState=InitialStates(6)  SwitchingTimes="[ 1/60  5/60 ]"  External=on  BreakerResistance=1e-4  SnubberResistance=1e6  SnubberCapacitance=inf  Measurements=None  MoreParameters=off  NoBreakLoop=off
      settings: SourceProductBaseCode=PS
  "Sw6 " : spsBreakerLib/Breaker  InitialState=InitialStates(7)  SwitchingTimes="[ 1/60  5/60 ]"  External=on  BreakerResistance=1e-6  SnubberResistance=1e8  SnubberCapacitance=inf  Measurements=None  MoreParameters=off  NoBreakLoop=off
      settings: SourceProductBaseCode=PS
  "Sw7 " : spsBreakerLib/Breaker  InitialState=InitialStates(8)  SwitchingTimes="[ 1/60  5/60 ]"  External=on  BreakerResistance=1e-6  SnubberResistance=1e68  SnubberCapacitance=inf  Measurements=None  MoreParameters=off  NoBreakLoop=off
      settings: SourceProductBaseCode=PS
  "Sw8 " : spsBreakerLib/Breaker  InitialState=InitialStates(9)  SwitchingTimes="[ 1/60  5/60 ]"  External=on  BreakerResistance=1e-6  SnubberResistance=1e8  SnubberCapacitance=inf  Measurements=None  MoreParameters=off  NoBreakLoop=off
      settings: SourceProductBaseCode=PS
  Sw9 : spsBreakerLib/Breaker  InitialState=InitialStates(10)  SwitchingTimes="[ 1/60  5/60 ]"  External=on  BreakerResistance=1e-6  SnubberResistance=1e8  SnubberCapacitance=inf  Measurements=None  MoreParameters=off  NoBreakLoop=off
      settings: SourceProductBaseCode=PS
  SwR1 : spsBreakerLib/Breaker  InitialState=1  SwitchingTimes="[ 1/60  5/60 ]"  External=on  BreakerResistance=1e-6  SnubberResistance=Rtransfer  SnubberCapacitance=inf  Measurements=None  MoreParameters=off  NoBreakLoop=off
      settings: SourceProductBaseCode=PS
  SwR2 : spsBreakerLib/Breaker  InitialState=1  SwitchingTimes="[ 1/60  5/60 ]"  External=on  BreakerResistance=1e-6  SnubberResistance=Rtransfer  SnubberCapacitance=inf  Measurements=None  MoreParameters=off  NoBreakLoop=off
      settings: SourceProductBaseCode=PS
  Tapped Winding Inversion : Subsystem
  Tap20 : PMIOPort  Side=Right
  Tap19 : PMIOPort  Port=2  Side=Right
  Tap18 : PMIOPort  Port=3  Side=Right
  Tap17 : PMIOPort  Port=4  Side=Right
  Tap16 : PMIOPort  Port=5  Side=Right
  Tap15 : PMIOPort  Port=6  Side=Right
  Tap14 : PMIOPort  Port=7  Side=Right
  Tap13 : PMIOPort  Port=8  Side=Right
  Tap12 : PMIOPort  Port=9  Side=Right
  Tap11 : PMIOPort  Port=10  Side=Right
  Tap10 : PMIOPort  Port=11  Side=Right
  Tap9 : PMIOPort  Port=12  Side=Right
  Tap8 : PMIOPort  Port=13  Side=Right
  Tap7 : PMIOPort  Port=14  Side=Right
  Tap6 : PMIOPort  Port=15  Side=Right
  Tap5 : PMIOPort  Port=16  Side=Right
  Tap4 : PMIOPort  Port=17  Side=Right
  Tap3 : PMIOPort  Port=18  Side=Right
  Tap2 : PMIOPort  Port=19  Side=Right
  Tap1 : PMIOPort  Port=20  Side=Right
  Tap0 : PMIOPort  Port=21  Side=Right
  W2+ : PMIOPort  Port=22  Side=Right
  Out : PMIOPort  Port=23  Side=Left
  wires:
  Demux/9 -> "Sw8 "/1
  Demux/8 -> "Sw7 "/1
  Demux/7 -> Display/1, "Sw6 "/1
  Demux/6 -> "Sw5 "/1
  Demux/5 -> "Sw4 "/1
  Demux/4 -> "Sw3 "/1
  Demux/3 -> "Sw2 "/1
  Demux/2 -> "Sw1 "/1
  Demux/1 -> "Sw0 "/1
  [SwInversion] -> Tapped Winding Inversion/1(Inv)
  [SwTransfer] -> SwR2/1, SwR1/1
  [SwSelect] -> Demux/1, Display1/1
  Demux/10 -> Sw9/1
  Demux/11 -> Sw10/1
  Demux/12 -> Sw11/1
  Demux/13 -> Sw12/1
  Demux/14 -> Sw13/1
  Demux/15 -> Sw14/1
  Demux/16 -> Sw15/1
  Demux/17 -> Sw16/1
  Demux/18 -> Sw17/1
  Demux/19 -> Sw18/1
  Demux/20 -> Sw19/1
  Demux/21 -> Sw20/1
  connections:
  "Sw0 "/LConn1 -- Tap0/RConn1 -- Tapped Winding Inversion/LConn2
  Tap1/RConn1 -- "Sw1 "/LConn1
  Tap2/RConn1 -- "Sw2 "/LConn1
  Tap6/RConn1 -- "Sw6 "/LConn1
  Tap4/RConn1 -- "Sw4 "/LConn1
  Tap5/RConn1 -- "Sw5 "/LConn1
  SwR1/RConn1 -- Tapped Winding Inversion/LConn1 -- SwR2/RConn1
  SwR2/LConn1 -- Sw19/RConn1 -- Sw17/RConn1 -- Sw15/RConn1 -- Sw13/RConn1 -- Sw11/RConn1 -- Sw9/RConn1 -- "Sw7 "/RConn1 -- "Sw5 "/RConn1 -- "Sw3 "/RConn1 -- "Sw1 "/RConn1
  Tapped Winding Inversion/RConn1 -- Out/RConn1
  W2+/RConn1 -- Tapped Winding Inversion/RConn2
  "Sw6 "/RConn1 -- "Sw4 "/RConn1 -- "Sw2 "/RConn1 -- "Sw0 "/RConn1 -- Sw20/RConn1 -- Sw18/RConn1 -- Sw16/RConn1 -- Sw14/RConn1 -- Sw12/RConn1 -- Sw10/RConn1 -- "Sw8 "/RConn1 -- SwR1/LConn1
  Tap3/RConn1 -- "Sw3 "/LConn1
  Tap8/RConn1 -- "Sw8 "/LConn1
  Tap7/RConn1 -- "Sw7 "/LConn1
  Tap9/RConn1 -- Sw9/LConn1
  Tap10/RConn1 -- Sw10/LConn1
  Tap11/RConn1 -- Sw11/LConn1
  Tap13/RConn1 -- Sw13/LConn1
  Tap12/RConn1 -- Sw12/LConn1
  Tap14/RConn1 -- Sw14/LConn1
  Tap15/RConn1 -- Sw15/LConn1
  Tap16/RConn1 -- Sw16/LConn1
  Tap17/RConn1 -- Sw17/LConn1
  Tap18/RConn1 -- Sw18/LConn1
  Tap19/RConn1 -- Sw19/LConn1
  Tap20/RConn1 -- Sw20/LConn1

== system ANS_GFM_short_term/OLTC/Subsystem ==
  note: A) Open the Three-Phase OLTC Transformer  mask (use Edit/Edit mask)
      |      In Initialization section, modify 1st line as below:
      |                   NumberOfTaps=10;
      |
      | B) Open the TransformerA block dialog box inside the Three-Phase OLTC Transformer (use Edit/Look under mask)
      |      and change the 'Number of Taps' parameter  from 7 to 9 (adding two intermediate taps on upper left winding (winding 1)).
      |
      | C) Open the  OLTCA block inside the Three-Phase OLTC Transformer (use Edit/Look under mask) and make the following changes:
      |       1) Open the dialog box of the Demux block and change the parameter  'Number of outputs' from 9 to 11.
      |       2) Add 2 switches labeled Sw9 and Sw10 (duplicate Sw8 block); Position these two blocks on top of Sw8 block.
      |       3) Open the dialog box of Sw9 and Sw10 blocks and change the  parameter "Initial state" as follows:
      |              Sw9 --> InitialState(10)
      |              Sw10-->InitialState(11)
      |      4) Add two connection ports labeled  respectively Tap9 and Tap10 (duplicate Tap8 block). Position these two blocks on top of Tap8 block.
      |      5) Renumber ALL connection ports as follows:
      |         Open dialog box of each connection port and change  'Port number' and  'Port location' parameters as in the table below.
      |         (all port locations should be set to  'right' except for 'Out' port which must be 'left')
      |         Start the renumbering with the top port  labeled Tap10.
      |
      |            Port           Port          Port
      |            label       number   location
      |           ---------    -----------    -----------
      |            Tap10       1               right
      |            Tap9         2               right
      |            .....            ......              .......
      |            Tap 1       11               right
      |            Tap 0       12               right
      |            W2+         13               right
      |            Out           14               left
      |
      |     6) Connect terminal 1 of Sw9 and Sw10 respectively to ports labeled Tap10 (port #1)  and Tap9  (port #2)
      |     7) Connect terminal 2 of Sw9 and Sw10 respectively to nodes labeled R2 and R1
      |     8) Close the OLTCA block.
      |
      | D)  Connect the Tap10, Tap9 ...Tap0 connectors of OLTCA respectively to  1+, 1.1,   ... 1 connectors of tapped winding of TransformerA.
      |
      | E)  Cut  the OLTCB and OLTCC blocks and replace them with a duplicate of OLTCA block.  Rename these two blocks OLTCB and OLTCC.
      |
      | F)  Cut  the TransformerB and TransformerC blocks and replace them with a duplicate of TransformerA block. Rename these two blocks TransformerB and TransformerC.
      |
      | G) Make connections between OLTC to Transformer for  phases B and C as for phase A.
      |
      | H) Ckeck that the secondary windings of  the three transformers are connected in Delta (D1)
  note: The following procedure explains how to increase the number of taps from 8 (17 OLTC positions)  to 10  (21 OLTC positions)
      |    If you want to decrease the number of taps, follow the reverse procedure (Change 'add' to ' cut'  and skip step C3).

== system ANS_GFM_short_term/OLTC/Voltage regulator ==
  Vmes (pu) : Inport
  Ready : Inport  Port=2
  RegOn : Inport  Port=3
  Dead Zone : DeadZone  LowerValue=-DeadBand/2  UpperValue=+DeadBand/2  SaturateOnIntegerOverflow=on
  Logical Operator : Logic  AllPortsSameDT=off
  Logical Operator1 : Logic  AllPortsSameDT=off
  MyDelay1 : Subsystem
  MyDelay2 : Subsystem
  Relational Operator : RelationalOperator  Operator=>  RndMeth=Nearest
  Relational Operator1 : RelationalOperator  Operator=<  RndMeth=Nearest
  Sum : Sum  Inputs=|+-  SaturateOnIntegerOverflow=on
  Switch : Switch  Threshold=1.5  SaturateOnIntegerOverflow=on
  Transport Delay : TransportDelay  DelayTime=Ts  InitialOutput=1
  Vref : Constant  Value=Vref
  Vref1 : Constant  Value=0
  Vref2 : Constant  Value=0
  Vref3 : Constant  Value=0
  Up : Outport  VectorParamsAs1DForOutWhenUnconnected=off
  Down : Outport  Port=2  VectorParamsAs1DForOutWhenUnconnected=off
  wires:
  Vref2/1 -> Switch/3
  RegOn/1 -> Switch/2
  Switch/1 -> Dead Zone/1
  Sum/1 -> Switch/1
  Vref/1 -> Sum/1
  Vmes (pu)/1 -> Sum/2
  Dead Zone/1 -> Relational Operator1/1, Relational Operator/1
  Vref1/1 -> Relational Operator/2
  Relational Operator/1 -> Logical Operator/1
  Ready/1 -> Transport Delay/1
  Transport Delay/1 -> Logical Operator1/1, Logical Operator/2
  Relational Operator1/1 -> Logical Operator1/2
  Logical Operator1/1 -> MyDelay1/1(in)
  Vref3/1 -> Relational Operator1/2
  MyDelay2/1(out) -> Up/1
  MyDelay1/1(out) -> Down/1
  Logical Operator/1 -> MyDelay2/1(in)

== system ANS_GFM_short_term/OLTC for load flow/ OLTC Control ==
  note: The 2 resistors are in operation during TransferTime/3
  note: Tap changer Mechanical Delay= TapSelectionTime
  Up : Inport
  Down : Inport  Port=2
  Abs1 : Abs  SaturateOnIntegerOverflow=on
  Constant : Constant  Value=TapVector
  Edge Detector : spsEdgeDetectorLib/Edge Detector  model=Rising  ic=0  Ts=0
      settings: SourceProductBaseCode=PS
  Logical Operator : Logic  Operator=NOT  AllPortsSameDT=off
  Monostable1 : spsMonostableLib/Monostable  EdgeDetect=Rising  PulseDuration=TransferTime  ic=1  Ts=0
      settings: SourceProductBaseCode=PS
  Off Delay : spsOnDelayLib/On Delay  DelayType=Off delay  delay=2*TransferTime/3  ic=InitialStates  Ts=0
      settings: SourceProductBaseCode=PS
  On Delay : spsOnDelayLib/On Delay  DelayType=On delay  delay=TransferTime/3  ic=1  Ts=0
      settings: SourceProductBaseCode=PS
  Relational Operator : RelationalOperator  Operator===  RndMeth=Nearest
  S-R Flip-Flop : simulink_extras/Flip Flops/S-R Flip-Flop  initial_condition=InitialTap>=0
  Set Reset : Subsystem
  Tap Changer Control : Subsystem  mask(Tap Changer Control){MinMaxTap=[-NumberOfTaps  +NumberOfTaps], InitialPosition=InitialTap, MecDelay=TapSelectionTime}
      mask prompts: MinMaxTap "Minimum and maximum tap number [ Min  Max ] :"; InitialPosition "Initial tap position"; MecDelay "Mechanical delay time"
      mask init:
      | if MecDelay<=0,
      | 	MecDelay=1/60;
      | end
  Terminator1 : Terminator
  Tap : Outport  VectorParamsAs1DForOutWhenUnconnected=off
  SwSelect : Outport  Port=2  VectorParamsAs1DForOutWhenUnconnected=off
  SwTr : Outport  Port=3  VectorParamsAs1DForOutWhenUnconnected=off
  SwInv : Outport  Port=4  VectorParamsAs1DForOutWhenUnconnected=off
  Ready : Outport  Port=5  VectorParamsAs1DForOutWhenUnconnected=off
  wires:
  Constant/1 -> Relational Operator/2
  Logical Operator/1 -> SwTr/1
  Down/1 -> Tap Changer Control/2(Down)
  Up/1 -> Tap Changer Control/1(Up)
  Relational Operator/1 -> On Delay/1
  Monostable1/1 -> Logical Operator/1
  Tap Changer Control/1(TapNo) -> Tap/1, Edge Detector/1, Set Reset/1(Tap), Abs1/1
  Tap Changer Control/2(Ready) -> Ready/1
  S-R Flip-Flop/2 -> Terminator1/1
  Edge Detector/1 -> Monostable1/1
  S-R Flip-Flop/1 -> SwInv/1
  Abs1/1 -> Relational Operator/1
  On Delay/1 -> Off Delay/1
  Off Delay/1 -> SwSelect/1
  Set Reset/1(Set) -> S-R Flip-Flop/1
  Set Reset/2(Reset) -> S-R Flip-Flop/2
